simulink model "Pre_rot_trif"  (R2017a)
settings: Solver=VariableStepAuto  StartTime=0.0  StopTime=1/30  RelTol=1e-3
libraries: fl_lib x40, nesl_utility x7
settings Model: Creator=gabriel  LastModifiedBy=gabriel

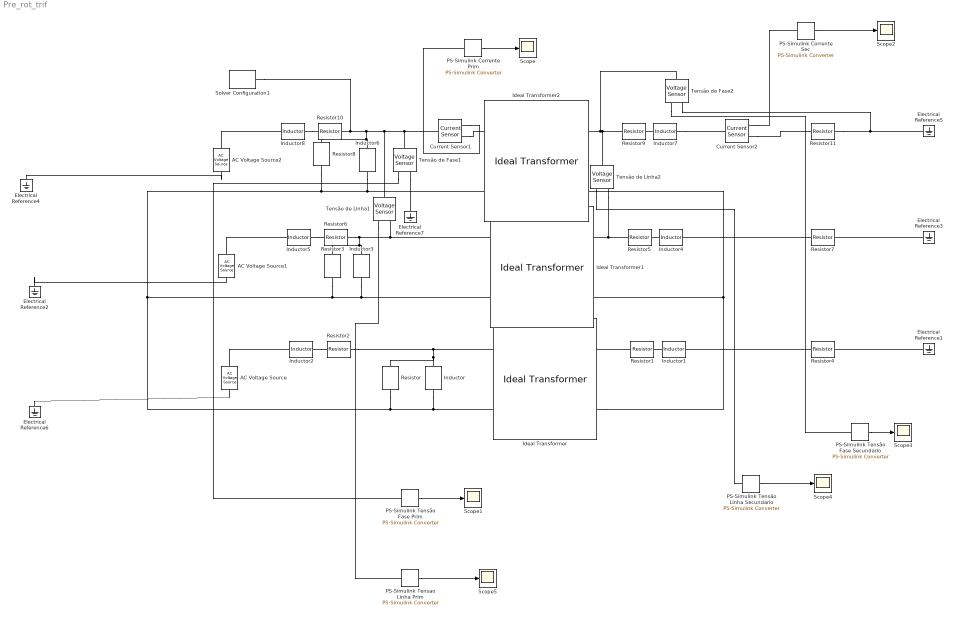
== system Pre_rot_trif ==
  AC Voltage Source : fl_lib/Electrical/Electrical Sources/AC Voltage Source  amp=220*1.4 V  shift=0 deg  frequency=60 Hz  omega=0 rad/s
  AC Voltage Source1 : fl_lib/Electrical/Electrical Sources/AC Voltage Source  amp=220*1.4 V  shift=120 deg  frequency=60 Hz  omega=0 rad/s
  AC Voltage Source2 : fl_lib/Electrical/Electrical Sources/AC Voltage Source  amp=220*1.4 V  shift=240 deg  frequency=60 Hz  omega=0 rad/s
  Current Sensor1 : fl_lib/Electrical/Electrical Sensors/Current Sensor
  Current Sensor2 : fl_lib/Electrical/Electrical Sensors/Current Sensor
  Electrical Reference{1..7} (7 alike) : fl_lib/Electrical/Electrical Elements/Electrical Reference
  Ideal Transformer : fl_lib/Electrical/Electrical Elements/Ideal Transformer  n=2  i1_specify=off  i1_priority=None  i1=0 A  i1_nominal_specify=off  i1_nominal_unit=A  i1_nominal_value=1  v1_specify=off  v1_priority=None  v1=0 V  v1_nominal_specify=off  v1_nominal_unit=V  v1_nominal_value=1  i2_specify=off  i2_priority=None  i2=0 A  i2_nominal_specify=off  i2_nominal_unit=A  i2_nominal_value=1  v2_specify=off  v2_priority=None  v2=0 V  v2_nominal_specify=off  v2_nominal_unit=V  v2_nominal_value=1
      settings: SourceProductName=Simscape  SourceProductBaseCode=SS
  Ideal Transformer1 : fl_lib/Electrical/Electrical Elements/Ideal Transformer  n=2  i1_specify=off  i1_priority=None  i1=0 A  i1_nominal_specify=off  i1_nominal_unit=A  i1_nominal_value=1  v1_specify=off  v1_priority=None  v1=0 V  v1_nominal_specify=off  v1_nominal_unit=V  v1_nominal_value=1  i2_specify=off  i2_priority=None  i2=0 A  i2_nominal_specify=off  i2_nominal_unit=A  i2_nominal_value=1  v2_specify=off  v2_priority=None  v2=0 V  v2_nominal_specify=off  v2_nominal_unit=V  v2_nominal_value=1
      settings: SourceProductName=Simscape  SourceProductBaseCode=SS
  Ideal Transformer2 : fl_lib/Electrical/Electrical Elements/Ideal Transformer  n=2  i1_specify=off  i1_priority=None  i1=0 A  i1_nominal_specify=off  i1_nominal_unit=A  i1_nominal_value=1  v1_specify=off  v1_priority=None  v1=0 V  v1_nominal_specify=off  v1_nominal_unit=V  v1_nominal_value=1  i2_specify=off  i2_priority=None  i2=0 A  i2_nominal_specify=off  i2_nominal_unit=A  i2_nominal_value=1  v2_specify=off  v2_priority=None  v2=0 V  v2_nominal_specify=off  v2_nominal_unit=V  v2_nominal_value=1
      settings: SourceProductName=Simscape  SourceProductBaseCode=SS
  Inductor : fl_lib/Electrical/Electrical Elements/Inductor  l=2000/(2*pi*60) H  r=0 Ohm  g=1e-9 1/Ohm  i_specify=off  i_priority=None  i=0 A  i_nominal_specify=off  i_nominal_unit=A  i_nominal_value=1  v_specify=off  v_priority=None  v=0 V  v_nominal_specify=off  v_nominal_unit=V  v_nominal_value=1  i_L_specify=off  i_L_priority=High  i_L=0 A  i_L_nominal_specify=off  i_L_nominal_unit=A  i_L_nominal_value=1
  Inductor{1..2,4..5,7..8} (6 alike) : fl_lib/Electrical/Electrical Elements/Inductor  l=100/(2*pi*60) H  r=0 Ohm  g=1e-9 1/Ohm  i_specify=off  i_priority=None  i=0 A  i_nominal_specify=off  i_nominal_unit=A  i_nominal_value=1  v_specify=off  v_priority=None  v=0 V  v_nominal_specify=off  v_nominal_unit=V  v_nominal_value=1  i_L_specify=off  i_L_priority=High  i_L=0 A  i_L_nominal_specify=off  i_L_nominal_unit=A  i_L_nominal_value=1
  Inductor3 : fl_lib/Electrical/Electrical Elements/Inductor  l=2000/(2*pi*60) H  r=0 Ohm  g=1e-9 1/Ohm  i_specify=off  i_priority=None  i=0 A  i_nominal_specify=off  i_nominal_unit=A  i_nominal_value=1  v_specify=off  v_priority=None  v=0 V  v_nominal_specify=off  v_nominal_unit=V  v_nominal_value=1  i_L_specify=off  i_L_priority=High  i_L=0 A  i_L_nominal_specify=off  i_L_nominal_unit=A  i_L_nominal_value=1
  Inductor6 : fl_lib/Electrical/Electrical Elements/Inductor  l=2000/(2*pi*60) H  r=0 Ohm  g=1e-9 1/Ohm  i_specify=off  i_priority=None  i=0 A  i_nominal_specify=off  i_nominal_unit=A  i_nominal_value=1  v_specify=off  v_priority=None  v=0 V  v_nominal_specify=off  v_nominal_unit=V  v_nominal_value=1  i_L_specify=off  i_L_priority=High  i_L=0 A  i_L_nominal_specify=off  i_L_nominal_unit=A  i_L_nominal_value=1
  "PS-Simulink Tensão Fase Prim " : nesl_utility/PS-Simulink Converter  PhysicalDomain=network_engine_domain  SubClassName=ps_output  LeftPortType=input  RightPortType=output  PseudoPeriodic=off  Frequencies=[]  Unit=1  AffineConversion=off
  "PS-Simulink Tensão Fase Secundario " : nesl_utility/PS-Simulink Converter  PhysicalDomain=network_engine_domain  SubClassName=ps_output  LeftPortType=input  RightPortType=output  PseudoPeriodic=off  Frequencies=[]  Unit=1  AffineConversion=off
  PS-Simulink Tensão Linha Secundario : nesl_utility/PS-Simulink Converter  PhysicalDomain=network_engine_domain  SubClassName=ps_output  LeftPortType=input  RightPortType=output  PseudoPeriodic=off  Frequencies=[]  Unit=1  AffineConversion=off
  "PS-Simulink Corrente Prim " : nesl_utility/PS-Simulink Converter  PhysicalDomain=network_engine_domain  SubClassName=ps_output  LeftPortType=input  RightPortType=output  PseudoPeriodic=off  Frequencies=[]  Unit=1  AffineConversion=off
  "PS-Simulink Corrente Sec " : nesl_utility/PS-Simulink Converter  PhysicalDomain=network_engine_domain  SubClassName=ps_output  LeftPortType=input  RightPortType=output  PseudoPeriodic=off  Frequencies=[]  Unit=1  AffineConversion=off
  "PS-Simulink Tensao Linha Prim " : nesl_utility/PS-Simulink Converter  PhysicalDomain=network_engine_domain  SubClassName=ps_output  LeftPortType=input  RightPortType=output  PseudoPeriodic=off  Frequencies=[]  Unit=1  AffineConversion=off
  Resistor : fl_lib/Electrical/Electrical Elements/Resistor  R=1000 Ohm  i_specify=off  i_priority=None  i=0 A  i_nominal_specify=off  i_nominal_unit=A  i_nominal_value=1  v_specify=off  v_priority=None  v=0 V  v_nominal_specify=off  v_nominal_unit=V  v_nominal_value=1
  Resistor{1..2,5..6,9..10} (6 alike) : fl_lib/Electrical/Electrical Elements/Resistor  R=10 Ohm  i_specify=off  i_priority=None  i=0 A  i_nominal_specify=off  i_nominal_unit=A  i_nominal_value=1  v_specify=off  v_priority=None  v=0 V  v_nominal_specify=off  v_nominal_unit=V  v_nominal_value=1
  Resistor11 : fl_lib/Electrical/Electrical Elements/Resistor  R=200 Ohm  i_specify=off  i_priority=None  i=0 A  i_nominal_specify=off  i_nominal_unit=A  i_nominal_value=1  v_specify=off  v_priority=None  v=0 V  v_nominal_specify=off  v_nominal_unit=V  v_nominal_value=1
  Resistor3 : fl_lib/Electrical/Electrical Elements/Resistor  R=1000 Ohm  i_specify=off  i_priority=None  i=0 A  i_nominal_specify=off  i_nominal_unit=A  i_nominal_value=1  v_specify=off  v_priority=None  v=0 V  v_nominal_specify=off  v_nominal_unit=V  v_nominal_value=1
  Resistor4 : fl_lib/Electrical/Electrical Elements/Resistor  R=200 Ohm  i_specify=off  i_priority=None  i=0 A  i_nominal_specify=off  i_nominal_unit=A  i_nominal_value=1  v_specify=off  v_priority=None  v=0 V  v_nominal_specify=off  v_nominal_unit=V  v_nominal_value=1
  Resistor7 : fl_lib/Electrical/Electrical Elements/Resistor  R=200 Ohm  i_specify=off  i_priority=None  i=0 A  i_nominal_specify=off  i_nominal_unit=A  i_nominal_value=1  v_specify=off  v_priority=None  v=0 V  v_nominal_specify=off  v_nominal_unit=V  v_nominal_value=1
  Resistor8 : fl_lib/Electrical/Electrical Elements/Resistor  R=1000 Ohm  i_specify=off  i_priority=None  i=0 A  i_nominal_specify=off  i_nominal_unit=A  i_nominal_value=1  v_specify=off  v_priority=None  v=0 V  v_nominal_specify=off  v_nominal_unit=V  v_nominal_value=1
  Scope{,1..5} (6 alike) : Scope
  Solver Configuration1 : nesl_utility/Solver Configuration  PhysicalDomain=network_engine_domain  SubClassName=solver  LeftPortType=input  RightPortType=generic  Accelerate=off  Tones=[]  Harmonics=[]  SimulateNoise=off  Profile=off  UseLocalSampling=off  EnableSwitchedLinearOptims=on  FrequencyDomain=off  UseCCode=off  RelTol=0.001  AbsTol=1e-06  MinStep=1e-09  ToWorkspace=off  RevertToSquareIcSolve=off  NumHomotopyIterations=100  PhasorMode=off  PhasorModeNumHarmonics=1  OverrideAbsTol=off  DoDC=off  ResidualTolerance=1e-09  UseLocalSolver=off  LocalSolverChoice=NE_BACKWARD_EULER_ADVANCER  LocalSolverSampleTime=0.001  DoFixedCost=off  MaxNonlinIter=3  MaxModeIter=2  LinearAlgebra=Sparse  DelaysMemoryBudget=1024  AutomaticFiltering=on  FilteringTimeConstant=0.001
  Tensão de Fase1 : fl_lib/Electrical/Electrical Sensors/Voltage Sensor
  Tensão de Fase2 : fl_lib/Electrical/Electrical Sensors/Voltage Sensor
  Tensão de Linha1 : fl_lib/Electrical/Electrical Sensors/Voltage Sensor
  Tensão de Linha2 : fl_lib/Electrical/Electrical Sensors/Voltage Sensor
  wires:
  "PS-Simulink Corrente Prim "/1 -> Scope/1
  "PS-Simulink Tensão Fase Prim "/1 -> Scope1/1
  "PS-Simulink Corrente Sec "/1 -> Scope2/1
  "PS-Simulink Tensão Fase Secundario "/1 -> Scope3/1
  PS-Simulink Tensão Linha Secundario/1 -> Scope4/1
  "PS-Simulink Tensao Linha Prim "/1 -> Scope5/1
  connections:
  Resistor1/LConn1 -- Ideal Transformer/RConn1
  Resistor2/RConn1 -- Inductor/LConn1 -- Resistor/LConn1 -- Ideal Transformer/LConn1
  Resistor4/LConn1 -- Inductor1/RConn1
  AC Voltage Source/LConn1 -- Inductor2/LConn1
  Inductor1/LConn1 -- Resistor1/RConn1
  Inductor2/RConn1 -- Resistor2/LConn1
  Resistor6/RConn1 -- Inductor3/LConn1 -- Resistor3/LConn1 -- Ideal Transformer1/LConn1 -- Tensão de Linha1/RConn2
  Resistor7/LConn1 -- Inductor4/RConn1
  Inductor5/RConn1 -- Resistor6/LConn1
  Resistor5/LConn1 -- Tensão de Linha2/RConn2 -- Ideal Transformer1/RConn1
  AC Voltage Source1/LConn1 -- Inductor5/LConn1
  Inductor4/LConn1 -- Resistor5/RConn1
  Resistor10/RConn1 -- Solver Configuration1/RConn1 -- Inductor6/LConn1 -- Resistor8/LConn1 -- Current Sensor1/LConn1 -- Tensão de Fase1/LConn1 -- Tensão de Linha1/LConn1
  Current Sensor2/RConn2 -- Resistor11/LConn1
  Inductor8/RConn1 -- Resistor10/LConn1
  Resistor9/LConn1 -- Tensão de Fase2/LConn1 -- Ideal Transformer2/RConn1 -- Tensão de Linha2/LConn1
  AC Voltage Source2/LConn1 -- Inductor8/LConn1
  Inductor7/LConn1 -- Resistor9/RConn1
  AC Voltage Source2/RConn1 -- Electrical Reference4/LConn1
  Electrical Reference2/LConn1 -- AC Voltage Source1/RConn1
  AC Voltage Source/RConn1 -- Electrical Reference6/LConn1
  Ideal Transformer2/LConn2 -- Inductor6/RConn1 -- Inductor/RConn1 -- Ideal Transformer/LConn2 -- Resistor/RConn1 -- Ideal Transformer1/LConn2 -- Inductor3/RConn1 -- Resistor3/RConn1 -- Resistor8/RConn1
  Resistor11/RConn1 -- Tensão de Fase2/RConn2 -- Electrical Reference5/LConn1
  Electrical Reference3/LConn1 -- Resistor7/RConn1
  Electrical Reference1/LConn1 -- Resistor4/RConn1
  Ideal Transformer2/RConn2 -- Ideal Transformer/RConn2 -- Ideal Transformer1/RConn2
  Tensão de Fase1/RConn2 -- Electrical Reference7/LConn1
  Current Sensor1/RConn2 -- Ideal Transformer2/LConn1
  Inductor7/RConn1 -- Current Sensor2/LConn1
  Current Sensor1/RConn1 -- "PS-Simulink Corrente Prim "/LConn1
  Tensão de Fase1/RConn1 -- "PS-Simulink Tensão Fase Prim "/LConn1
  Tensão de Linha1/RConn1 -- "PS-Simulink Tensao Linha Prim "/LConn1
  Current Sensor2/RConn1 -- "PS-Simulink Corrente Sec "/LConn1
  Tensão de Linha2/RConn1 -- PS-Simulink Tensão Linha Secundario/LConn1
  Tensão de Fase2/RConn1 -- "PS-Simulink Tensão Fase Secundario "/LConn1
